simulink model "loop"  (R2019b)
settings: Solver=VariableStepAuto  StartTime=0.0  StopTime=1.5  RelTol=1e-3  EnableMultiTasking=on
settings Model: PauseTimes=100  Creator=kwono  LastModifiedBy=SAMSUNG PC
settings DataIOCC: ReturnWorkspaceOutputs=off
settings OptimizationCC: LifeSpan=inf
settings DebuggingCC: SFUnexpectedBacktrackingDiag=warning  SFNoUnconditionalDefaultTransitionDiag=warning  ArithmeticOperatorsInVariantConditions=warning
settings SFSimCC: SimUseLocalCustomCode=off  CustomCodeUndefinedFunction=UseInterfaceOnly
settings RTWCC: RTWUseLocalCustomCode=off
settings CodeAppCC: StateflowObjectComments=on
settings GRTTargetCC: TargetLangStandard=C89/C90 (ANSI)  GeneratePreprocessorConditionals=Disable all
settings ConfigComp: CovMetricSettings=dw  CovHtmlReporting=on  CovSaveCumulativeToWorkspaceVar=on  CovSaveSingleToWorkspaceVar=on  CovExternalEMLEnable=off

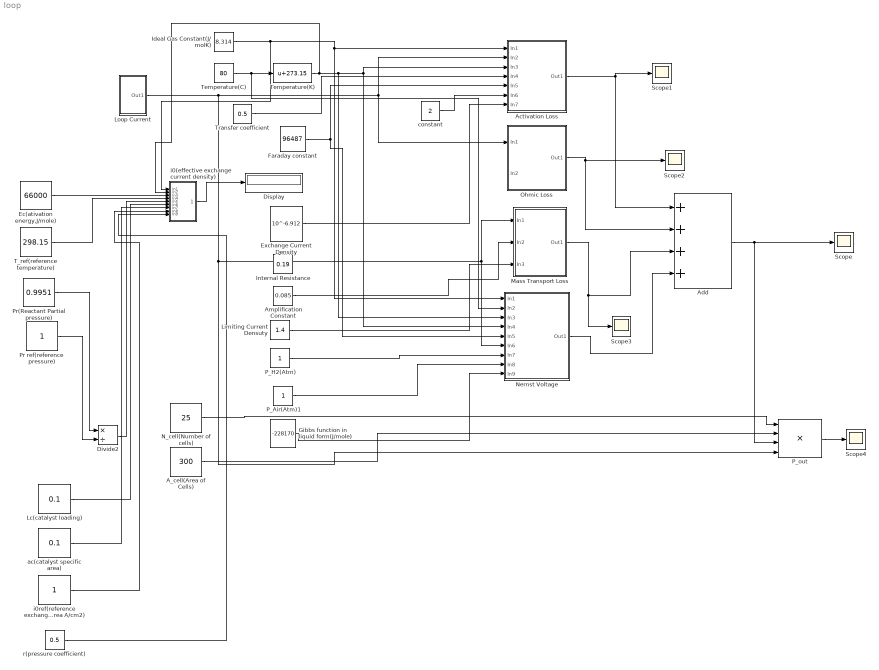
== system loop ==
  A_cell(Area of Cells) : Constant  Value=300
  Activation Loss : Subsystem
  Add : Sum  Inputs=++++
  Amplification Constant : Constant  Value=0.085
  Display : Display
  Divide2 : Product  Inputs=*/
  Ec(ativation energy,J/mole) : Constant  Value=66000
  Exchange Current Density : Constant  Value=10^-6.912
  Faraday constant : Constant  Value=96487
  Gibbs function in liquid form(J/mole) : Constant  Value=-228170
  Ideal Gas Constant(J/molK) : Constant  Value=8.314
  Internal Resistance : Constant  Value=0.19
  Lc(catalyst loading) : Constant  Value=0.1
  Limiting Current Densuty : Constant  Value=1.4
  Loop Current : Subsystem
  Mass Transport Loss : Subsystem
  N_cell(Number of cells) : Constant  Value=25
  Nernst Voltage : Subsystem
  Ohmic Loss : Subsystem
  P_Air(Atm)1 : Constant
  P_H2(Atm) : Constant
  P_out : Product  Inputs=4
  Pr ref(reference pressure) : Constant
  Pr(Reactant Partial pressure) : Constant  Value=0.9951
  Scope{,1..4} (5 alike) : Scope
  T_ref(reference temperature) : Constant  Value=298.15
  Temperature(C) : Constant  Value=80
  Temperature(K) : Fcn  Expr=u+273.15
  Transfer coefficient : Constant  Value=0.5
  ac(catalyst specific area) : Constant  Value=0.1
  constant : Constant  Value=2
  i0(effective exchange current density) : Subsystem
  i0ref(reference exchange current density per unit catalyst surface area A/cm2) : Constant
  r(pressure coefficient) : Constant  Value=0.5
  wires:
  Temperature(C)/1 -> Nernst Voltage/2(In2), Temperature(K)/1
  Transfer coefficient/1 -> Activation Loss/4(In4)
  constant/1 -> Activation Loss/6(In6)
  Exchange Current Density/1 -> Activation Loss/7(In7)
  Amplification Constant/1 -> Mass Transport Loss/2(In2)
  Limiting Current Densuty/1 -> Mass Transport Loss/3(In3)
  Activation Loss/1(Out1) -> Add/1, Scope1/1
  Ohmic Loss/1(Out1) -> Add/2, Scope2/1
  Mass Transport Loss/1(Out1) -> Scope3/1, Add/3
  Add/1 -> P_out/3, Scope/1
  Faraday constant/1 -> Nernst Voltage/5(In5), Activation Loss/5(In5)
  Ideal Gas Constant(J/molK)/1 -> i0(effective exchange current density)/1(In1), Nernst Voltage/1(In1), Activation Loss/1(In1)
  Loop Current/1(Out1) -> Activation Loss/2(In2), Ohmic Loss/1(In1), Nernst Voltage/6(In6), Mass Transport Loss/1(In1), P_out/4
  Temperature(K)/1 -> i0(effective exchange current density)/2(In2), Nernst Voltage/3(In3), Nernst Voltage/4(In4), Activation Loss/3(In3)
  P_H2(Atm)/1 -> Nernst Voltage/7(In7)
  P_Air(Atm)1/1 -> Nernst Voltage/8(In8)
  Gibbs function in liquid form(J/mole)/1 -> Nernst Voltage/9(In9)
  Nernst Voltage/1(Out1) -> Add/4
  N_cell(Number of cells)/1 -> P_out/1
  A_cell(Area of Cells)/1 -> P_out/2
  P_out/1 -> Scope4/1
  Pr ref(reference pressure)/1 -> Divide2/2
  Pr(Reactant Partial pressure)/1 -> Divide2/1
  Ec(ativation energy,J/mole)/1 -> i0(effective exchange current density)/3(In3)
  T_ref(reference temperature)/1 -> i0(effective exchange current density)/4(In4)
  Divide2/1 -> i0(effective exchange current density)/5(In5)
  Lc(catalyst loading)/1 -> i0(effective exchange current density)/6(In6)
  ac(catalyst specific area)/1 -> i0(effective exchange current density)/7(In7)
  i0ref(reference exchange current density per unit catalyst surface area A/cm2)/1 -> i0(effective exchange current density)/8(In8)
  r(pressure coefficient)/1 -> i0(effective exchange current density)/9(In9)
  i0(effective exchange current density)/1(Out1) -> Display/1

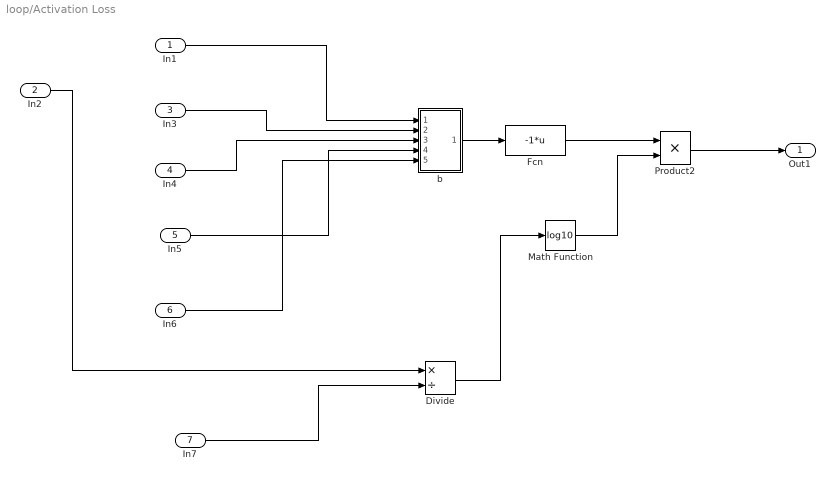
== system loop/Activation Loss ==
  In1 : Inport
  In2 : Inport  Port=2
  In3 : Inport  Port=3
  In4 : Inport  Port=4
  In5 : Inport  Port=5
  In6 : Inport  Port=6
  In7 : Inport  Port=7
  Divide : Product  Inputs=*/
  Fcn : Fcn  Expr=-1*u
  Math Function : Math  Operator=log10  SaturateOnIntegerOverflow=on
  Product2 : Product
  b : Subsystem
  Out1 : Outport
  wires:
  b/1(Out1) -> Fcn/1
  Product2/1 -> Out1/1
  Fcn/1 -> Product2/1
  In7/1 -> Divide/2
  Divide/1 -> Math Function/1
  Math Function/1 -> Product2/2
  In6/1 -> b/5(In5)
  In4/1 -> b/3(In3)
  In1/1 -> b/1(In1)
  In3/1 -> b/2(In2)
  In5/1 -> b/4(In4)
  In2/1 -> Divide/1

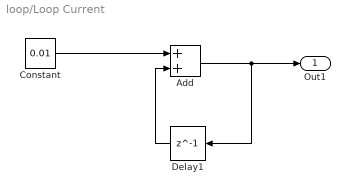
== system loop/Loop Current ==
  Add : Sum
  Constant : Constant  Value=0.01  OutMax=[2]
  Delay1 : Delay  DelayLength=1  InitialCondition=0  SampleTime=0.01
  Out1 : Outport
  wires:
  Constant/1 -> Add/1
  Delay1/1 -> Add/2
  Add/1 -> Out1/1, Delay1/1

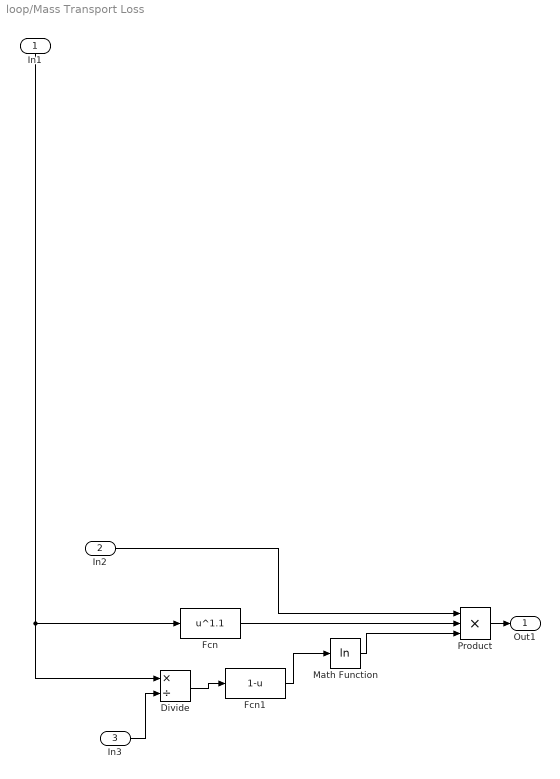
== system loop/Mass Transport Loss ==
  In1 : Inport
  In2 : Inport  Port=2
  In3 : Inport  Port=3
  Divide : Product  Inputs=*/
  Fcn : Fcn  Expr=u^1.1
  Fcn1 : Fcn  Expr=1-u
  Math Function : Math  Operator=log  SaturateOnIntegerOverflow=on
  Product : Product  Inputs=3
  Out1 : Outport
  wires:
  Fcn/1 -> Product/2
  In3/1 -> Divide/2
  Divide/1 -> Fcn1/1
  Fcn1/1 -> Math Function/1
  Math Function/1 -> Product/3
  In2/1 -> Product/1
  Product/1 -> Out1/1
  In1/1 -> Divide/1, Fcn/1

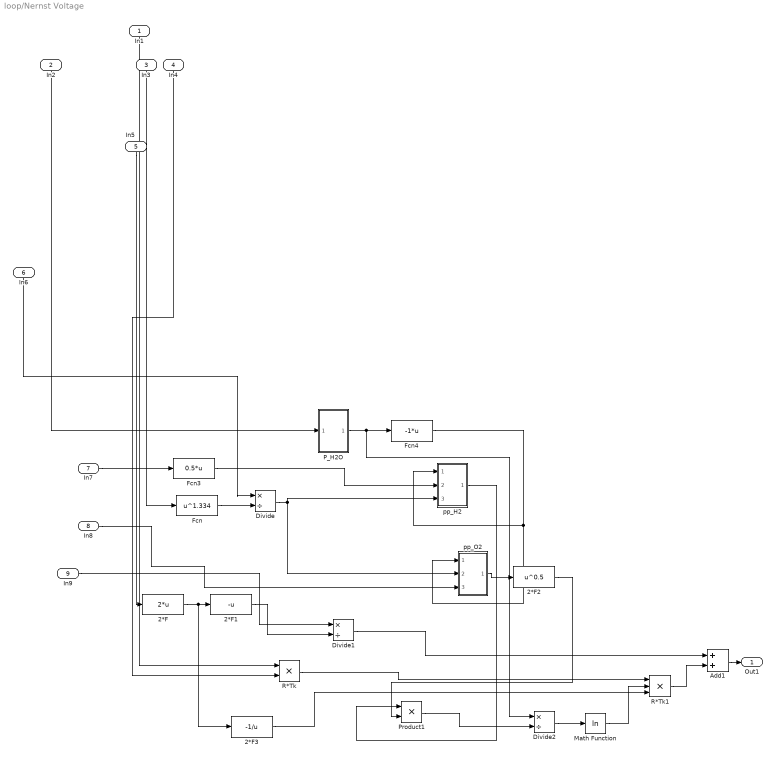
== system loop/Nernst Voltage ==
  In1 : Inport
  In2 : Inport  Port=2
  In3 : Inport  Port=3
  In4 : Inport  Port=4
  In5 : Inport  Port=5
  In6 : Inport  Port=6
  In7 : Inport  Port=7
  In8 : Inport  Port=8
  In9 : Inport  Port=9
  2*F : Fcn  Expr=2*u
  2*F1 : Fcn  Expr=-u
  2*F2 : Fcn  Expr=u^0.5
  2*F3 : Fcn  Expr=-1/u
  Add1 : Sum
  Divide : Product  Inputs=*/
  Divide1 : Product  Inputs=*/
  Divide2 : Product  Inputs=*/
  Fcn : Fcn  Expr=u^1.334
  Fcn3 : Fcn  Expr=0.5*u
  Fcn4 : Fcn  Expr=-1*u
  Math Function : Math  Operator=log  SaturateOnIntegerOverflow=on
  P_H2O : Subsystem
  Product1 : Product
  R*Tk : Product
  R*Tk1 : Product  Inputs=3
  pp_H2 : Subsystem
  pp_O2 : Subsystem
  Out1 : Outport
  wires:
  P_H2O/1(Out1) -> Divide2/1, Fcn4/1
  In7/1 -> Fcn3/1
  Fcn4/1 -> pp_O2/1(In1), pp_H2/1(In1)
  Fcn3/1 -> pp_H2/2(In2)
  Add1/1 -> Out1/1
  In6/1 -> Divide/1
  Product1/1 -> Divide2/2
  pp_H2/1(Out1) -> Product1/1
  2*F/1 -> 2*F3/1, 2*F1/1
  Divide/1 -> pp_O2/2(In2), pp_H2/3(In3)
  Fcn/1 -> Divide/2
  R*Tk1/1 -> Add1/2
  Divide1/1 -> Add1/1
  Divide2/1 -> Math Function/1
  pp_O2/1(Out1) -> 2*F2/1
  In5/1 -> 2*F/1
  In3/1 -> Fcn/1
  In4/1 -> R*Tk/2
  In2/1 -> P_H2O/1(In1)
  In1/1 -> R*Tk/1
  Math Function/1 -> R*Tk1/2
  R*Tk/1 -> R*Tk1/1
  In9/1 -> Divide1/1
  2*F1/1 -> Divide1/2
  2*F2/1 -> Product1/2
  2*F3/1 -> R*Tk1/3
  In8/1 -> pp_O2/3(In3)

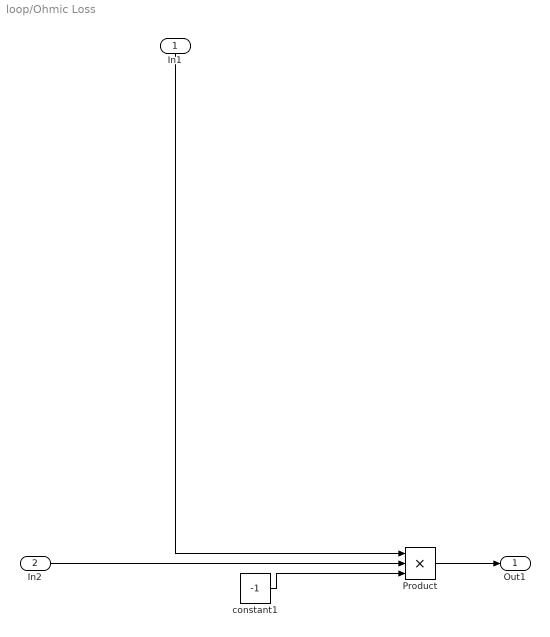
== system loop/Ohmic Loss ==
  In1 : Inport
  In2 : Inport  Port=2
  Product : Product  Inputs=3
  constant1 : Constant  Value=-1
  Out1 : Outport
  wires:
  In1/1 -> Product/1
  In2/1 -> Product/2
  constant1/1 -> Product/3
  Product/1 -> Out1/1

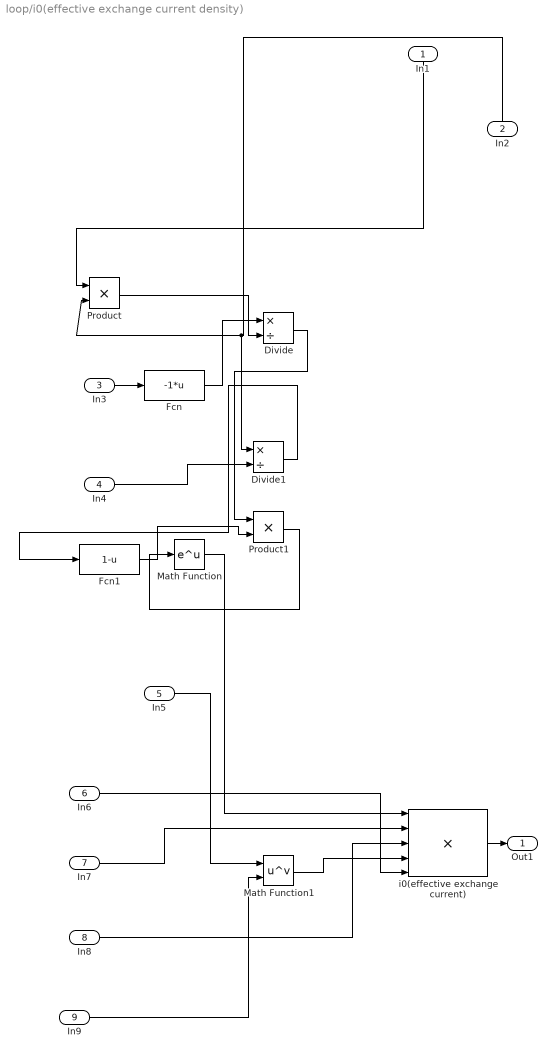
== system loop/i0(effective exchange current density) ==
  In1 : Inport
  In2 : Inport  Port=2
  In3 : Inport  Port=3
  In4 : Inport  Port=4
  In5 : Inport  Port=5
  In6 : Inport  Port=6
  In7 : Inport  Port=7
  In8 : Inport  Port=8
  In9 : Inport  Port=9
  Divide : Product  Inputs=*/
  Divide1 : Product  Inputs=*/
  Fcn : Fcn  Expr=-1*u
  Fcn1 : Fcn  Expr=1-u
  Math Function : Math  SaturateOnIntegerOverflow=on
  Math Function1 : Math  Operator=pow  SaturateOnIntegerOverflow=on
  Product : Product
  Product1 : Product
  i0(effective exchange current) : Product  Inputs=5
  Out1 : Outport
  wires:
  In8/1 -> i0(effective exchange current)/3
  Divide1/1 -> Fcn1/1
  Product/1 -> Divide/2
  Math Function/1 -> i0(effective exchange current)/1
  Product1/1 -> Math Function/1
  Math Function1/1 -> i0(effective exchange current)/4
  In9/1 -> Math Function1/2
  Fcn/1 -> Divide/1
  Fcn1/1 -> Product1/2
  In7/1 -> i0(effective exchange current)/2
  In6/1 -> i0(effective exchange current)/5
  In1/1 -> Product/1
  i0(effective exchange current)/1 -> Out1/1
  In2/1 -> Divide1/1, Product/2
  Divide/1 -> Product1/1
  In3/1 -> Fcn/1
  In4/1 -> Divide1/2
  In5/1 -> Math Function1/1

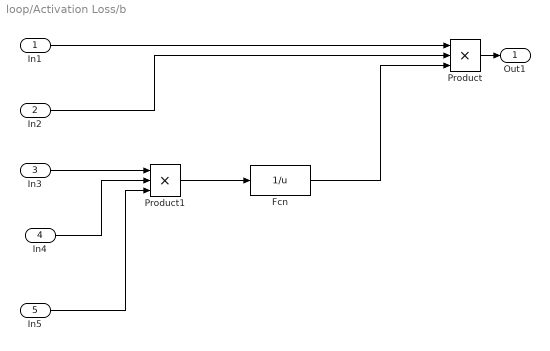
== system loop/Activation Loss/b ==
  In1 : Inport
  In2 : Inport  Port=2
  In3 : Inport  Port=3
  In4 : Inport  Port=4
  In5 : Inport  Port=5
  Fcn : Fcn  Expr=1/u
  Product : Product  Inputs=3
  Product1 : Product  Inputs=3
  Out1 : Outport
  wires:
  In1/1 -> Product/1
  In4/1 -> Product1/2
  In2/1 -> Product/2
  In3/1 -> Product1/1
  Product/1 -> Out1/1
  In5/1 -> Product1/3
  Product1/1 -> Fcn/1
  Fcn/1 -> Product/3

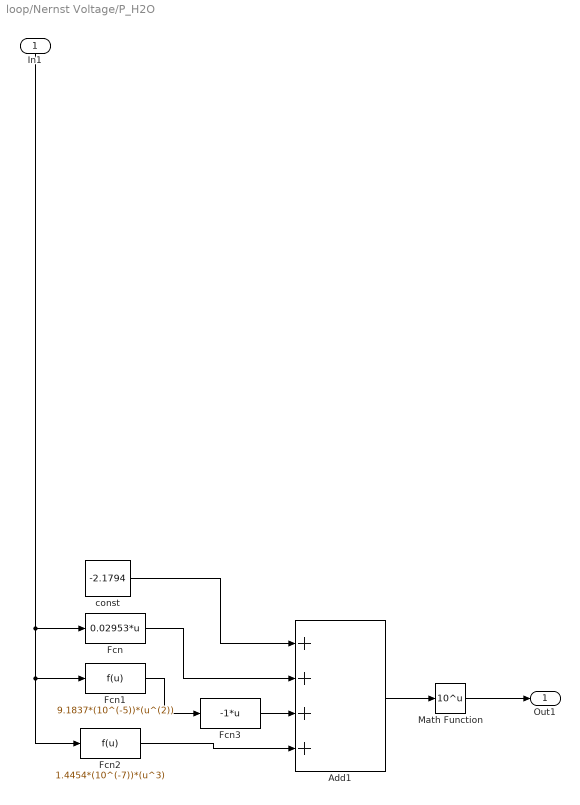
== system loop/Nernst Voltage/P_H2O ==
  In1 : Inport
  Add1 : Sum  Inputs=++++
  Fcn : Fcn  Expr=0.02953*u
  Fcn1 : Fcn  Expr=9.1837*(10^(-5))*(u^(2))
  Fcn2 : Fcn  Expr=1.4454*(10^(-7))*(u^3)
  Fcn3 : Fcn  Expr=-1*u
  Math Function : Math  Operator=10^u  SaturateOnIntegerOverflow=on
  const : Constant  Value=-2.1794
  Out1 : Outport
  wires:
  In1/1 -> Fcn2/1, Fcn1/1, Fcn/1
  Add1/1 -> Math Function/1
  Fcn1/1 -> Fcn3/1
  Fcn/1 -> Add1/2
  const/1 -> Add1/1
  Fcn3/1 -> Add1/3
  Math Function/1 -> Out1/1
  Fcn2/1 -> Add1/4

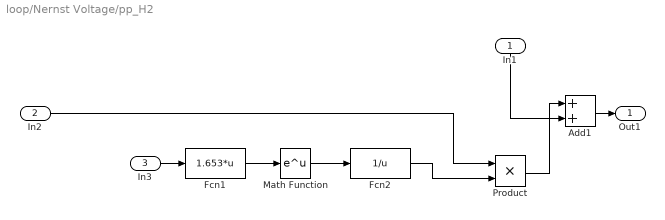
== system loop/Nernst Voltage/pp_H2 ==
  In1 : Inport
  In2 : Inport  Port=2
  In3 : Inport  Port=3
  Add1 : Sum
  Fcn1 : Fcn  Expr=1.653*u
  Fcn2 : Fcn  Expr=1/u
  Math Function : Math  SaturateOnIntegerOverflow=on
  Product : Product
  Out1 : Outport
  wires:
  Math Function/1 -> Fcn2/1
  In2/1 -> Product/1
  In1/1 -> Add1/2
  In3/1 -> Fcn1/1
  Add1/1 -> Out1/1
  Fcn2/1 -> Product/2
  Product/1 -> Add1/1
  Fcn1/1 -> Math Function/1

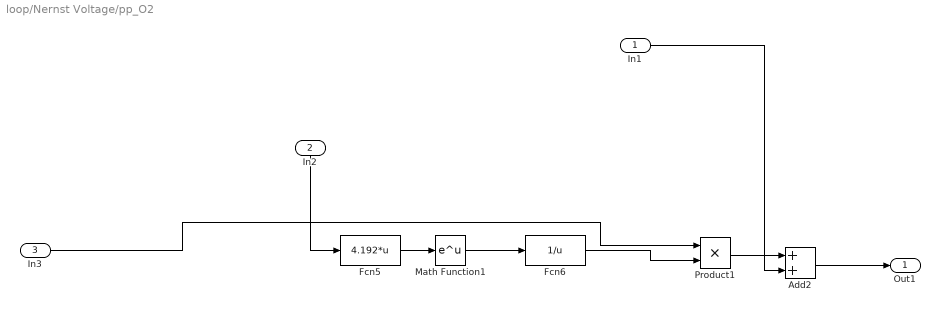
== system loop/Nernst Voltage/pp_O2 ==
  In1 : Inport
  In2 : Inport  Port=2
  In3 : Inport  Port=3
  Add2 : Sum
  Fcn5 : Fcn  Expr=4.192*u
  Fcn6 : Fcn  Expr=1/u
  Math Function1 : Math  SaturateOnIntegerOverflow=on
  Product1 : Product
  Out1 : Outport
  wires:
  Product1/1 -> Add2/1
  Add2/1 -> Out1/1
  In3/1 -> Product1/1
  Math Function1/1 -> Fcn6/1
  In2/1 -> Fcn5/1
  In1/1 -> Add2/2
  Fcn5/1 -> Math Function1/1
  Fcn6/1 -> Product1/2
